simulink library "speedgoatlib_evse"  (R2024b)
settings: Solver=VariableStepAuto  StartTime=0.0  StopTime=10.0  RelTol=1e-3
undefined symbols (not defined in the file): sg_ev_charging_read_m, sg_ev_charging_write_m, sg_ev_isolation_read_m, sg_ev_parameter_read_m, sg_ev_parameter_write_m, sg_ev_precharge_read_m, sg_ev_precharge_write_m, sg_ev_status_m, sg_ev_stop_read_m, sg_ev_stop_write_m, sg_ev_welding_read_m, sg_ev_welding_write_m, sg_evse_charging_read_m, sg_evse_charging_write_m, sg_evse_isolation_read_m, sg_evse_isolation_write_m, sg_evse_parameter_read_m, sg_evse_parameter_write_m, sg_evse_precharge_read_m, sg_evse_precharge_write_m, sg_evse_status_m, sg_evse_stop_read_m, sg_evse_stop_write_m, sg_evse_welding_read_m, sg_evse_welding_write_m
libraries: speedgoatlib_mqtt x199, simulink x39, $bdroot x24
(part 1 of 8)
settings Model: Creator=timo.straessle  LastModifiedBy=speedgoat\jenkins
settings OptimizationCC: ReuseModelBlockBuffer=off
settings RTWCC: GPUComputeCapability=3.5
settings ConfigComp: CovBoundaryAbsTol=1.0e-5

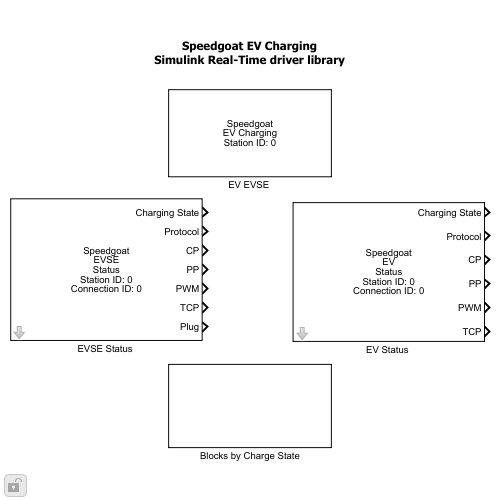
[thumbnail: Simulink's stored preview of the top-level diagram]
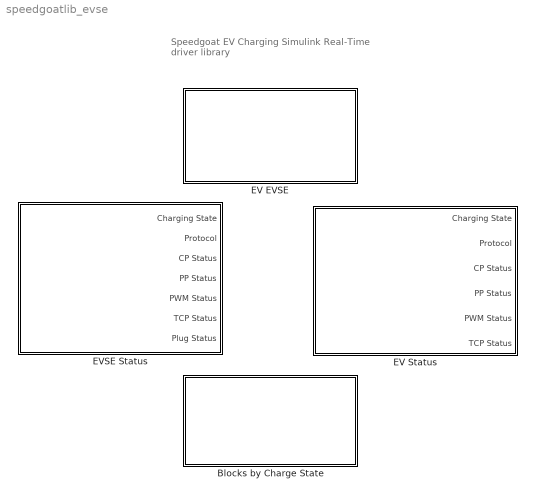
== system speedgoatlib_evse ==
  note: Speedgoat EV Charging
      | Simulink Real-Time driver library
  Blocks by Charge State : Subsystem
  "EV EVSE " : Subsystem  mask(EV_EVSE){}
      settings: OpenFcn=sg_evse.openFcnConfig;
      mask Help: eval('sg.utils.help.show(''io_main/refentry_ref_ev_evse'');')
      mask Display: disp('Speedgoat\nEV Charging\nStation ID: 0');
  "EV Status " : Subsystem  InitFcn=sg_ev_status_m.runInitFcn();  mask(status_EV){parClientId=0, parConnectionId=0, parSampleTime=-1}
      mask prompts: parClientId "Station ID"; parConnectionId "Connection ID"; parSampleTime "Sample Time"
      mask help: Speedgoat Driver Block<br>EV - Status<br><br>&copy; 2007 - 2026, Speedgoat GmbH, <a href="matlab: web('www.speedgoat.com','-browser');">www.speedgoat.com</a>
      mask init:
      | sg_ev_status_m.runMaskInit();
      mask Help: eval('sg.utils.help.show(''io_main/refentry_ref_ev_status'');')
      mask DialogControl Container6 Prompt: Main
      mask DialogControl Container3 Prompt: Connection Setup
      mask Display: disp('Speedgoat\nEV\nStatus\nStation ID: 0\nConnection ID: 0');port_label('output',1,'Charging State');port_label('output',2,'Protocol');port_label('output',3,'CP');port_label('output',4,'PP');port_label('output',5,'PWM');port_label('output',6,'TCP');
  "EVSE Status " : Subsystem  InitFcn=sg_evse_status_m.runInitFcn();  mask(status_EVSE){parClientId=0, parConnectionId=0, parSampleTime=-1}
      mask prompts: parClientId "Station ID"; parConnectionId "Connection ID"; parSampleTime "Sample Time"
      mask help: Speedgoat Driver Block<br>EVSE - Status<br><br>&copy; 2007 - 2026, Speedgoat GmbH, <a href="matlab: web('www.speedgoat.com','-browser');">www.speedgoat.com</a>
      mask init:
      | sg_evse_status_m.runMaskInit();
      mask Help: eval('sg.utils.help.show(''io_main/refentry_ref_evse_status'');')
      mask DialogControl Container6 Prompt: Main
      mask DialogControl Container3 Prompt: Connection Setup
      mask Display: disp('Speedgoat\nEVSE\nStatus\nStation ID: 0\nConnection ID: 0');port_label('output',1,'Charging State');port_label('output',2,'Protocol');port_label('output',3,'CP');port_label('output',4,'PP');port_label('output',5,'PWM');port_label('output',6,'TCP');port_label('output',7,'Plug');

== system speedgoatlib_evse/Blocks by Charge State ==
  note: EV
  note: EVSE
  "EV Charging Read " : Subsystem  InitFcn=sg_ev_charging_read_m.runInitFcn();  mask(charging_read_EV){parClientId=0, parConnectionId=0, parSampleTime=-1}
      mask prompts: parClientId "Station ID"; parConnectionId "Connection ID"; parSampleTime "Sample Time"
      mask help: Speedgoat Driver Block<br>EV - Charging<br><br>&copy; 2007 - 2026, Speedgoat GmbH, <a href="matlab: web('www.speedgoat.com','-browser');">www.speedgoat.com</a>
      mask init:
      | sg_ev_charging_read_m.runMaskInit();
      mask Help: eval('sg.utils.help.show(''io_main/refentry_ref_ev_charging_read'');')
      mask DialogControl Container6 Prompt: Main
      mask DialogControl Container3 Prompt: Connection Setup
      mask Display: disp('Speedgoat\nEV\nCharging\nRead\nStation ID: 0\nConnection ID: 0');port_label('output',1,'EVSE Present Voltage');port_label('output',2,'EVSE Present Current');port_label('output',3,'EVSE Current Limit Achieved');port_label('output',4,'EVSE Voltage Limit Achieved');port_label('output',5,'EVSE Power Limit Achieved');port_label('output',6,'EVSE Max Voltage Limit');port_label('output',7,'EVSE Max Current Limit');port_label('output',8,'EVSE Max Power Limit');
  "EV Charging Write " : Subsystem  InitFcn=sg_ev_charging_write_m.runInitFcn();  mask(charging_write_EV){parClientId=0, parConnectionId=0, parSampleTime=-1, parEnReadyToChargeState=on, parEnChargingProfileTupleId=on, parEnChargeReady=on, parEnErrorCode=on, parEnRessSoc=on, parEnTargetVoltage=on, parEnTargetCurrent=on, parEnBulkChargingComplete=on, parEnChargingComplete=on, parEnRemainingTimeToBulkSoc=on, parEnRemainingTimeToFullSoc=on}
      mask prompts: parClientId "Station ID"; parConnectionId "Connection ID"; parSampleTime "Sample Time"; parEnReadyToChargeState "Ready to Charge State"; parEnChargingProfileTupleId "Charging Profile Tuple ID"; parEnChargeReady "Charge Ready"; parEnErrorCode "Errorcode"; parEnRessSoc "RESS SOC"; parEnTargetVoltage "Target Voltage"; parEnTargetCurrent "Target Current"; parEnBulkChargingComplete "Bulk Charging Complete"; parEnChargingComplete "Charging Complete"; parEnRemainingTimeToBulkSoc "Remaining Time to Bulk SOC"; parEnRemainingTimeToFullSoc "Remaining Time to Full SOC"
      mask help: Speedgoat Driver Block<br>EV - Charging<br><br>&copy; 2007 - 2026, Speedgoat GmbH, <a href="matlab: web('www.speedgoat.com','-browser');">www.speedgoat.com</a>
      mask init:
      | sg_ev_charging_write_m.runMaskInit();
      mask Help: eval('sg.utils.help.show(''io_main/refentry_ref_ev_charging_write'');')
      mask DialogControl Container6 Prompt: Main
      mask DialogControl Container3 Prompt: Connection Setup
      mask DialogControl Container10 Prompt: Enable/Disable Signals
      mask Display: disp('Speedgoat\nEV\nCharging\nWrite\nStation ID: 0\nConnection ID: 0');port_label('input',1,'Ready to Charge State');port_label('input',2,'Charging Profile Tuple ID');port_label('input',3,'Charge Ready');port_label('input',4,'Errorcode');port_label('input',5,'RESS SOC');port_label('input',6,'Target Voltage');port_label('input',7,'Target Current');port_label('input',8,'Bulk Charging Complete');port_label('input',9,'Charging Complete');port_label('input',10,'Remaining Time to Bulk SOC');port_label('input',11,'Remaining Time to Full SOC');
  "EV Isolation Read " : Subsystem  InitFcn=sg_ev_isolation_read_m.runInitFcn();  mask(isolation_read_EV){parClientId=0, parConnectionId=0, parSampleTime=-1}
      mask prompts: parClientId "Station ID"; parConnectionId "Connection ID"; parSampleTime "Sample Time"
      mask help: Speedgoat Driver Block<br>EV - Isolation<br><br>&copy; 2007 - 2026, Speedgoat GmbH, <a href="matlab: web('www.speedgoat.com','-browser');">www.speedgoat.com</a>
      mask init:
      | sg_ev_isolation_read_m.runMaskInit();
      mask Help: eval('sg.utils.help.show(''io_main/refentry_ref_ev_isolation_read'');')
      mask DialogControl Container6 Prompt: Main
      mask DialogControl Container3 Prompt: Connection Setup
      mask Display: disp('Speedgoat\nEV\nIsolation\nRead\nStation ID: 0\nConnection ID: 0');port_label('output',1,'EVSE Processing');port_label('output',2,'EVSE Isolationstatus');port_label('output',3,'EVSE Statuscode');
  "EV Isolation Write " : Subsystem  InitFcn=sg_ev_precharge_write_m.runInitFcn();  mask(isolation_write_EV){parClientId=0, parConnectionId=0, parSampleTime=-1, parEnReady=on, parEnErrorCode=on, parEnRessSoc=on}
      mask prompts: parClientId "Station ID"; parConnectionId "Connection ID"; parSampleTime "Sample Time"; parEnReady "Ready"; parEnErrorCode "Errorcode"; parEnRessSoc "RESS SOC"
      mask help: Speedgoat Driver Block<br>EV - Isolation<br><br>&copy; 2007 - 2026, Speedgoat GmbH, <a href="matlab: web('www.speedgoat.com','-browser');">www.speedgoat.com</a>
      mask init:
      | sg_ev_isolation_write_m.runMaskInit();
      mask Help: eval('sg.utils.help.show(''io_main/refentry_ref_ev_isolation_write'');')
      mask DialogControl Container6 Prompt: Main
      mask DialogControl Container3 Prompt: Connection Setup
      mask DialogControl Container10 Prompt: Enable/Disable Signals
      mask Display: disp('Speedgoat\nEV\nIsolation\nWrite\nStation ID: 0\nConnection ID: 0');port_label('input',1,'Ready');port_label('input',2,'Errorcode');port_label('input',3,'RESS SOC');
  "EV Parameter Read " : Subsystem  InitFcn=sg_ev_parameter_read_m.runInitFcn();  mask(parameter_read_EV){parClientId=0, parConnectionId=0, parSampleTime=-1}
      mask prompts: parClientId "Station ID"; parConnectionId "Connection ID"; parSampleTime "Sample Time"
      mask help: Speedgoat Driver Block<br>EV - Parameter Discovery<br><br>&copy; 2007 - 2026, Speedgoat GmbH, <a href="matlab: web('www.speedgoat.com','-browser');">www.speedgoat.com</a>
      mask init:
      | sg_ev_parameter_read_m.runMaskInit();
      mask Help: eval('sg.utils.help.show(''io_main/refentry_ref_ev_parameter_read'');')
      mask DialogControl Container6 Prompt: Main
      mask DialogControl Container3 Prompt: Connection Setup
      mask Display: disp('Speedgoat\nEV\nParameter Discovery\nRead\nStation ID: 0\nConnection ID: 0');port_label('output',1,'SA-Schedule: ID');port_label('output',2,'SA-Schedule: Start');port_label('output',3,'SA-Schedule: Duration');port_label('output',4,'SA-Schedule: PMax');port_label('output',5,'EVSE Max Voltage Limit');port_label('output',6,'EVSE Max Current Limit');port_label('output',7,'EVSE Max Power Limit');port_label('output',8,'EVSE Min Current Limit');port_label('output',9,'EVSE Min Voltage Limit');port_label('output',10,'EVSE Current Regulation Tolerance');port_label('output',11,'EVSE Peak Current Ripple');port_label('output',12,'EVSE Energy to be Delivered');port_label('output',13,'EVSE Notification Max Delay');port_label('output',14,'EVSE Notification');port_label('output',15,'EVSE Isolationstatus');port_label('output',16,'EVSE Statuscode');
  "EV Parameter Write " : Subsystem  InitFcn=sg_ev_parameter_write_m.runInitFcn();  mask(parameter_write_EV){parClientId=0, parConnectionId=0, parSampleTime=-1, parEnRequestedEnergyType=on, parEnDepartureTime=on, parEnMaxVoltageLimit=on, parEnMaxCurrentLimit=on, parEnMinCurrentLimit=on, parEnMaxPowerLimit=on, parEnReady=on, parEnErrorcode=on, parEnRessSoc=on, parEnEnergyCapacity=on, parEnEnergyRequest=on, parEnFullSoc=on, parEnBulkSoc=on}
      mask prompts: parClientId "Station ID"; parConnectionId "Connection ID"; parSampleTime "Sample Time"; parEnRequestedEnergyType "Requested Energy Type"; parEnDepartureTime "Departure Time"; parEnMaxVoltageLimit "Max Voltage Limit"; parEnMaxCurrentLimit "Max Current Limit"; parEnMinCurrentLimit "Min Current Limit"; parEnMaxPowerLimit "Max Power Limit"; parEnReady "Ready"; parEnErrorcode "Errorcode"; parEnRessSoc "RESS SOC"; parEnEnergyCapacity "Energy Capacity"; parEnEnergyRequest "Energy Request"; parEnFullSoc "Full SOC"; parEnBulkSoc "Bulk SOC"
      mask help: Speedgoat Driver Block<br>EV - Parameter Discovery<br><br>&copy; 2007 - 2026, Speedgoat GmbH, <a href="matlab: web('www.speedgoat.com','-browser');">www.speedgoat.com</a>
      mask init:
      | sg_ev_parameter_write_m.runMaskInit();
      mask Help: eval('sg.utils.help.show(''io_main/refentry_ref_ev_parameter_write'');')
      mask DialogControl Container6 Prompt: Main
      mask DialogControl Container3 Prompt: Connection Setup
      mask DialogControl Container10 Prompt: Enable/Disable Signals
      mask DialogControl Control2 Prompt: Uncheck unused signals to disable them and avoid sending out zeroes.
      mask Display: disp('Speedgoat\nEV\nParameter Discovery\nWrite\nStation ID: 0\nConnection ID: 0');port_label('input',1,'Requested Energy Type');port_label('input',2,'Departure Time');port_label('input',3,'Max Voltage Limit');port_label('input',4,'Max Current Limit');port_label('input',5,'Min Current Limit');port_label('input',6,'Max Power Limit');port_label('input',7,'Ready');port_label('input',8,'Errorcode');port_label('input',9,'RESS SOC');port_label('input',10,'Energy Capacity');port_label('input',11,'Energy Request');port_label('input',12,'Full SOC');port_label('input',13,'Bulk SOC');
  "EV Pre-Charge Read " : Subsystem  InitFcn=sg_ev_precharge_read_m.runInitFcn();  mask(precharge_read_EV){parClientId=0, parConnectionId=0, parSampleTime=-1}
      mask prompts: parClientId "Station ID"; parConnectionId "Connection ID"; parSampleTime "Sample Time"
      mask help: Speedgoat Driver Block<br>EV - Pre-Charge<br><br>&copy; 2007 - 2026, Speedgoat GmbH, <a href="matlab: web('www.speedgoat.com','-browser');">www.speedgoat.com</a>
      mask init:
      | sg_ev_precharge_read_m.runMaskInit();
      mask Help: eval('sg.utils.help.show(''io_main/refentry_ref_ev_precharge_read'');')
      mask DialogControl Container6 Prompt: Main
      mask DialogControl Container3 Prompt: Connection Setup
      mask Display: disp('Speedgoat\nEV\nPre-Charge\nRead\nStation ID: 0\nConnection ID: 0');port_label('output',1,'EVSE Isolationstatus');port_label('output',2,'EVSE Statuscode');port_label('output',3,'EVSE Present Voltage');
  "EV Pre-Charge Write " : Subsystem  InitFcn=sg_ev_precharge_write_m.runInitFcn();  mask(precharge_write_EV){parClientId=0, parConnectionId=0, parSampleTime=-1, parEnReady=on, parEnErrorCode=on, parEnRessSoc=on, parEnTargetVoltage=on, parEnTargetCurrent=on}
      mask prompts: parClientId "Station ID"; parConnectionId "Connection ID"; parSampleTime "Sample Time"; parEnReady "Ready"; parEnErrorCode "Errorcode"; parEnRessSoc "RESS SOC"; parEnTargetVoltage "Target Voltage"; parEnTargetCurrent "Target Current"
      mask help: Speedgoat Driver Block<br>EV - Pre-Charge<br><br>&copy; 2007 - 2026, Speedgoat GmbH, <a href="matlab: web('www.speedgoat.com','-browser');">www.speedgoat.com</a>
      mask init:
      | sg_ev_precharge_write_m.runMaskInit();
      mask Help: eval('sg.utils.help.show(''io_main/refentry_ref_ev_precharge_write'');')
      mask DialogControl Container6 Prompt: Main
      mask DialogControl Container3 Prompt: Connection Setup
      mask DialogControl Container10 Prompt: Enable/Disable Signals
      mask Display: disp('Speedgoat\nEV\nPre-Charge\nWrite\nStation ID: 0\nConnection ID: 0');port_label('input',1,'Ready');port_label('input',2,'Errorcode');port_label('input',3,'RESS SOC');port_label('input',4,'Target Voltage');port_label('input',5,'Target Current');
  "EV Setup " : Subsystem  mask(setup_EV){parClientId=0, parConnectionId=0, parClientIdentifier='speedgoat', parIpAddrStr='192.168.10.7', parSampleTime=-1, parTcpPort=1883, parRemoteIpAddrStr='192.168.10.9', parDepartureTime=3600*4, parMaxVoltageLimit=480, parMaxCurrentLimit=100, parMinCurrentLimit=5, parMaxPowerLimit=60000, parRessSoc=30, parEnergyCapacity=80000, parEnergyRequest=30000, parFullSoc=100, parBulkSoc=80}
      mask prompts: parClientId "Station ID"; parConnectionId "Connection ID"; parClientIdentifier "Client Identifier"; parIpAddrStr "Local IP Address"; parSampleTime "Sample Time"; parTcpPort "Remote TCP Port"; parRemoteIpAddrStr "Remote IP Address"; parDepartureTime "Departure Time [s]"; parMaxVoltageLimit "Max. Voltage Limit [V]"; parMaxCurrentLimit "Max. Current Limit [A]"; parMinCurrentLimit "Min. Current Limit [A]"; parMaxPowerLimit "Max. Power Limit [W]"; parRessSoc "RESS SOC"; parEnergyCapacity "Energy Capacity [Wh]"; parEnergyRequest "Energy Request [Wh]"; parFullSoc "Full SOC"; parBulkSoc "Bulk SOC"
      mask Help: eval('sg.utils.help.show(''io_main/refentry_ref_ev_setup'');')
      mask TypeOptions parDepartureTime: departureTime/Value
      mask TypeOptions parMaxVoltageLimit: maxVoltageLimit/Value
      mask TypeOptions parMaxCurrentLimit: maxCurrentLimit/Value
      mask TypeOptions parMinCurrentLimit: minCurrentLimit/Value
      mask TypeOptions parMaxPowerLimit: maxPowerLimit/Value
      mask TypeOptions parRessSoc: ressSoc/Value
      mask TypeOptions parEnergyCapacity: energyCapacity/Value
      mask TypeOptions parEnergyRequest: energyRequest/Value
      mask TypeOptions parFullSoc: fullSoc/Value
      mask TypeOptions parBulkSoc: bulkSoc/Value
      mask DialogControl Container6 Prompt: Main
      mask DialogControl Container3 Prompt: Connection Setup
      mask DialogControl Container8 Prompt: EV Board Setup
      mask DialogControl Container10 Prompt: Vehicle Configuration Parameters
      mask Display: disp('Speedgoat\nEV Setup\n');
  "EV Stop Read " : Subsystem  InitFcn=sg_ev_stop_read_m.runInitFcn();  mask(stop_read_EV){parClientId=0, parConnectionId=0, parSampleTime=-1}
      mask prompts: parClientId "Station ID"; parConnectionId "Connection ID"; parSampleTime "Sample Time"
      mask help: Speedgoat Driver Block<br>EV - Stop<br><br>&copy; 2007 - 2026, Speedgoat GmbH, <a href="matlab: web('www.speedgoat.com','-browser');">www.speedgoat.com</a>
      mask init:
      | sg_ev_stop_read_m.runMaskInit();
      mask Help: eval('sg.utils.help.show(''io_main/refentry_ref_ev_stop_read'');')
      mask DialogControl Container6 Prompt: Main
      mask DialogControl Container3 Prompt: Connection Setup
      mask Display: disp('Speedgoat\nEV\nStop\nRead\nStation ID: 0\nConnection ID: 0');port_label('output',1,'EVSE Stop Progress');port_label('output',2,'EVSE Processing');
  "EV Stop Write " : Subsystem  InitFcn=sg_ev_stop_write_m.runInitFcn();  mask(stop_write_EV){parClientId=0, parConnectionId=0, parSampleTime=-1, parEnStopProgress=on}
      mask prompts: parClientId "Station ID"; parConnectionId "Connection ID"; parSampleTime "Sample Time"; parEnStopProgress "Stop Progress"
      mask help: Speedgoat Driver Block<br>EV - Stop<br><br>&copy; 2007 - 2026, Speedgoat GmbH, <a href="matlab: web('www.speedgoat.com','-browser');">www.speedgoat.com</a>
      mask init:
      | sg_ev_stop_write_m.runMaskInit();
      mask Help: eval('sg.utils.help.show(''io_main/refentry_ref_ev_stop_write'');')
      mask DialogControl Container6 Prompt: Main
      mask DialogControl Container3 Prompt: Connection Setup
      mask DialogControl Container10 Prompt: Enable/Disable Signals
      mask Display: disp('Speedgoat\nEV\nStop\nWrite\nStation ID: 0\nConnection ID: 0');port_label('input',1,'Stop Progress');
  "EV Welding Read " : Subsystem  InitFcn=sg_ev_welding_read_m.runInitFcn();  mask(welding_read_EV){parClientId=0, parConnectionId=0, parSampleTime=-1}
      mask prompts: parClientId "Station ID"; parConnectionId "Connection ID"; parSampleTime "Sample Time"
      mask help: Speedgoat Driver Block<br>EV - Welding<br><br>&copy; 2007 - 2026, Speedgoat GmbH, <a href="matlab: web('www.speedgoat.com','-browser');">www.speedgoat.com</a>
      mask init:
      | sg_ev_welding_read_m.runMaskInit();
      mask Help: eval('sg.utils.help.show(''io_main/refentry_ref_ev_welding_read'');')
      mask DialogControl Container6 Prompt: Main
      mask DialogControl Container3 Prompt: Connection Setup
      mask Display: disp('Speedgoat\nEV\nWelding\nRead\nStation ID: 0\nConnection ID: 0');port_label('output',1,'EVSE Notification');port_label('output',2,'EVSE Isolationstatus');port_label('output',3,'EVSE Statuscode');port_label('output',4,'EVSE Present Voltage');
  "EV Welding Write " : Subsystem  InitFcn=sg_ev_welding_write_m.runInitFcn();  mask(welding_write_EV){parClientId=0, parConnectionId=0, parSampleTime=-1, parEnReady=on, parEnErrorCode=on, parEnRessSoc=on}
      mask prompts: parClientId "Station ID"; parConnectionId "Connection ID"; parSampleTime "Sample Time"; parEnReady "Ready"; parEnErrorCode "Errorcode"; parEnRessSoc "RESS SOC"
      mask help: Speedgoat Driver Block<br>EV - Welding<br><br>&copy; 2007 - 2026, Speedgoat GmbH, <a href="matlab: web('www.speedgoat.com','-browser');">www.speedgoat.com</a>
      mask init:
      | sg_ev_welding_write_m.runMaskInit();
      mask Help: eval('sg.utils.help.show(''io_main/refentry_ref_ev_welding_write'');')
      mask DialogControl Container6 Prompt: Main
      mask DialogControl Container3 Prompt: Connection Setup
      mask DialogControl Container10 Prompt: Enable/Disable Signals
      mask Display: disp('Speedgoat\nEV\nWelding\nWrite\nStation ID: 0\nConnection ID: 0');port_label('input',1,'Ready');port_label('input',2,'Errorcode');port_label('input',3,'RESS SOC');
  "EVSE Charging Read " : Subsystem  InitFcn=sg_evse_charging_read_m.runInitFcn();  mask(charging_read_EVSE){parClientId=0, parConnectionId=0, parSampleTime=-1}
      mask prompts: parClientId "Station ID"; parConnectionId "Connection ID"; parSampleTime "Sample Time"
      mask help: Speedgoat Driver Block<br>EVSE - Charging<br><br>&copy; 2007 - 2026, Speedgoat GmbH, <a href="matlab: web('www.speedgoat.com','-browser');">www.speedgoat.com</a>
      mask init:
      | sg_evse_charging_read_m.runMaskInit();
      mask Help: eval('sg.utils.help.show(''io_main/refentry_ref_evse_charging_read'');')
      mask DialogControl Container6 Prompt: Main
      mask DialogControl Container3 Prompt: Connection Setup
      mask Display: disp('Speedgoat\nEVSE\nCharging\nRead\nStation ID: 0\nConnection ID: 0');port_label('output',1,'EV Ready');port_label('output',2,'EV Errorcode');port_label('output',3,'EV RESS SOC');port_label('output',4,'EV Target Voltage');port_label('output',5,'EV Target Current');port_label('output',6,'EV Max Voltage Limit');port_label('output',7,'EV Max Current Limit');port_label('output',8,'EV Max Power Limit');port_label('output',9,'EV Bulk Charging Complete');port_label('output',10,'EV Charging Complete');port_label('output',11,'EV Time to Bulk SOC');port_label('output',12,'EV Time to Full SOC');
  "EVSE Charging Write " : Subsystem  InitFcn=sg_evse_charging_write_m.runInitFcn();  mask(charging_write_EVSE){parClientId=0, parConnectionId=0, parSampleTime=-1, parEnNotification=on, parEnIsolationStatus=on, parEnStatusCode=on, parEnPresentVoltage=on, parEnPresentCurrent=on, parEnCurrentLimitAchieved=on, parEnVoltageLimitAchieved=on, parEnPowerLimitAchieved=on, parEnMaxVoltageLimit=on, parEnMaxCurrentLimit=on, parEnMaxPowerLimit=on}
      mask prompts: parClientId "Station ID"; parConnectionId "Connection ID"; parSampleTime "Sample Time"; parEnNotification "Notification"; parEnIsolationStatus "Isolationstatus"; parEnStatusCode "Statuscode"; parEnPresentVoltage "Present Voltage"; parEnPresentCurrent "Present Current"; parEnCurrentLimitAchieved "Current Limit Achieved"; parEnVoltageLimitAchieved "Voltage Limit Achieved"; parEnPowerLimitAchieved "Power Limit Achieved"; parEnMaxVoltageLimit "Max Voltage Limit"; parEnMaxCurrentLimit "Max Current Limit"; parEnMaxPowerLimit "Max Power Limit"
      mask help: Speedgoat Driver Block<br>EVSE - Charging<br><br>&copy; 2007 - 2026, Speedgoat GmbH, <a href="matlab: web('www.speedgoat.com','-browser');">www.speedgoat.com</a>
      mask init:
      | sg_evse_charging_write_m.runMaskInit();
      mask Help: eval('sg.utils.help.show(''io_main/refentry_ref_evse_charging_write'');')
      mask DialogControl Container6 Prompt: Main
      mask DialogControl Container3 Prompt: Connection Setup
      mask DialogControl Container10 Prompt: Enable/Disable Signals
      mask Display: disp('Speedgoat\nEVSE\nCharging\nWrite\nStation ID: 0\nConnection ID: 0');port_label('input',1,'Notification');port_label('input',2,'Isolationstatus');port_label('input',3,'Statuscode');port_label('input',4,'Present Voltage');port_label('input',5,'Present Current');port_label('input',6,'Current Limit Achieved');port_label('input',7,'Voltage Limit Achieved');port_label('input',8,'Power Limit Achieved');port_label('input',9,'Max Voltage Limit');port_label('input',10,'Max Current Limit');port_label('input',11,'Max Power Limit');
  "EVSE Isolation Read " : Subsystem  InitFcn=sg_evse_isolation_read_m.runInitFcn();  mask(isolation_read_EVSE){parClientId=0, parConnectionId=0, parSampleTime=-1}
      mask prompts: parClientId "Station ID"; parConnectionId "Connection ID"; parSampleTime "Sample Time"
      mask help: Speedgoat Driver Block<br>EVSE - Isolation<br><br>&copy; 2007 - 2026, Speedgoat GmbH, <a href="matlab: web('www.speedgoat.com','-browser');">www.speedgoat.com</a>
      mask init:
      | sg_evse_isolation_read_m.runMaskInit();
      mask Help: eval('sg.utils.help.show(''io_main/refentry_ref_evse_isolation_read'');')
      mask DialogControl Container6 Prompt: Main
      mask DialogControl Container3 Prompt: Connection Setup
      mask Display: disp('Speedgoat\nEVSE\nIsolation\nRead\nStation ID: 0\nConnection ID: 0');port_label('output',1,'EV Ready');port_label('output',2,'EV Errorcode');port_label('output',3,'EV RESS SOC');
  "EVSE Isolation Write " : Subsystem  InitFcn=sg_evse_isolation_write_m.runInitFcn();  mask(isolation_write_EVSE){parClientId=0, parConnectionId=0, parSampleTime=-1, parEnEvseProcessing=on, parEnIsolationStatus=on, parEnStatusCode=on}
      mask prompts: parClientId "Station ID"; parConnectionId "Connection ID"; parSampleTime "Sample Time"; parEnEvseProcessing "EVSE Processing"; parEnIsolationStatus "Isolationstatus"; parEnStatusCode "Statuscode"
      mask help: Speedgoat Driver Block<br>EVSE - Isolation<br><br>&copy; 2007 - 2026, Speedgoat GmbH, <a href="matlab: web('www.speedgoat.com','-browser');">www.speedgoat.com</a>
      mask init:
      | sg_evse_isolation_write_m.runMaskInit();
      mask Help: eval('sg.utils.help.show(''io_main/refentry_ref_evse_isolation_write'');')
      mask DialogControl Container6 Prompt: Main
      mask DialogControl Container3 Prompt: Connection Setup
      mask DialogControl Container10 Prompt: Enable/Disable Signals
      mask Display: disp('Speedgoat\nEVSE\nIsolation\nWrite\nStation ID: 0\nConnection ID: 0');port_label('input',1,'EVSE Processing');port_label('input',2,'Isolationstatus');port_label('input',3,'Statuscode');
  "EVSE Parameter Read " : Subsystem  InitFcn=sg_evse_parameter_read_m.runInitFcn();  mask(parameter_read_EVSE){parClientId=0, parConnectionId=0, parSampleTime=-1}
      mask prompts: parClientId "Station ID"; parConnectionId "Connection ID"; parSampleTime "Sample Time"
      mask help: Speedgoat Driver Block<br>EVSE - Parameter Discovery<br><br>&copy; 2007 - 2026, Speedgoat GmbH, <a href="matlab: web('www.speedgoat.com','-browser');">www.speedgoat.com</a>
      mask init:
      | sg_evse_parameter_read_m.runMaskInit();
      mask Help: eval('sg.utils.help.show(''io_main/refentry_ref_evse_parameter_read'');')
      mask DialogControl Container6 Prompt: Main
      mask DialogControl Container3 Prompt: Connection Setup
      mask Display: disp('Speedgoat\nEVSE\nParameter Discovery\nRead\nStation ID: 0\nConnection ID: 0');port_label('output',1,'EV Requested Energy Type');port_label('output',2,'EV Departure Time');port_label('output',3,'EV Max Voltage Limit');port_label('output',4,'EV Max Current Limit');port_label('output',5,'EV Min Current Limit');port_label('output',6,'EV Max Power Limit');port_label('output',7,'EV Ready');port_label('output',8,'EV Errorcode');port_label('output',9,'EV RESS SOC');port_label('output',10,'EV Energy Capacity');port_label('output',11,'EV Energy Request');port_label('output',12,'EV Full SOC');port_label('output',13,'EV Bulk SOC');
  "EVSE Parameter Write " : Subsystem  InitFcn=sg_evse_parameter_write_m.runInitFcn();  mask(parameter_write_EVSE){parClientId=0, parConnectionId=0, parSampleTime=-1, parEnEvseProcessing=on, parEnSaScheduleList=on, parEnMaxVoltageLimit=on, parEnMaxCurrentLimit=on, parEnMaxPowerLimit=on, parEnMinVoltageLimit=on, parEnMinCurrentLimit=on, parEnCurrRegTol=on, parEnPeakCurrentRipple=on, parEnEnergyToBeDelivered=on, parEnNotificationMaxDelay=on, parEnNotification=on, parEnIsolationStatus=on, parEnStatusCode=on}
      mask prompts: parClientId "Station ID"; parConnectionId "Connection ID"; parSampleTime "Sample Time"; parEnEvseProcessing "EVSE Processing"; parEnSaScheduleList "SA-Schedule List"; parEnMaxVoltageLimit "Max Voltage Limit"; parEnMaxCurrentLimit "Max Current Limit"; parEnMaxPowerLimit "Max Power Limit"; parEnMinVoltageLimit "Min Voltage Limit"; parEnMinCurrentLimit "Min Current Limit"; parEnCurrRegTol "Current Regulation Tolerance"; parEnPeakCurrentRipple "Peak Current Ripple"; parEnEnergyToBeDelivered "Energy To Be Delivered"; parEnNotificationMaxDelay "Notification Max Delay"; parEnNotification "Notification"; parEnIsolationStatus "Isolationstatus"; parEnStatusCode "Statuscode"
      mask help: Speedgoat Driver Block<br>EVSE - Parameter Discovery<br><br>&copy; 2007 - 2026, Speedgoat GmbH, <a href="matlab: web('www.speedgoat.com','-browser');">www.speedgoat.com</a>
      mask init:
      | sg_evse_parameter_write_m.runMaskInit();
      mask Help: eval('sg.utils.help.show(''io_main/refentry_ref_evse_parameter_write'');')
      mask DialogControl Container6 Prompt: Main
      mask DialogControl Container3 Prompt: Connection Setup
      mask DialogControl Container10 Prompt: Enable/Disable Signals
      mask DialogControl Control2 Prompt: Uncheck unused signals to disable them and avoid sending out zeroes.
      mask Display: disp('Speedgoat\nEVSE\nParameter Discovery\nWrite\nStation ID: 0\nConnection ID: 0');port_label('input',1,'EVSE Processing');port_label('input',2,'SA-Schedule: ID');port_label('input',3,'SA-Schedule: Start');port_label('input',4,'SA-Schedule: Duration');port_label('input',5,'SA-Schedule: PMax');port_label('input',6,'Max Voltage Limit');port_label('input',7,'Max Current Limit');port_label('input',8,'Max Power Limit');port_label('input',9,'Min Voltage Limit');port_label('input',10,'Min Current Limit');port_label('input',11,'Current Regulation Tolerance');port_label('input',12,'Peak Current Ripple');port_label('input',13,'Energy to be Delivered');port_label('input',14,'Notification Max Delay');port_label('input',15,'Notification');port_label('input',16,'Isolationstatus');port_label('input',17,'Statuscode');
  "EVSE Pre-Charge Read " : Subsystem  InitFcn=sg_evse_precharge_read_m.runInitFcn();  mask(precharge_read_EVSE){parClientId=0, parConnectionId=0, parSampleTime=-1}
      mask prompts: parClientId "Station ID"; parConnectionId "Connection ID"; parSampleTime "Sample Time"
      mask help: Speedgoat Driver Block<br>EVSE - Pre-Charge<br><br>&copy; 2007 - 2026, Speedgoat GmbH, <a href="matlab: web('www.speedgoat.com','-browser');">www.speedgoat.com</a>
      mask init:
      | sg_evse_precharge_read_m.runMaskInit();
      mask Help: eval('sg.utils.help.show(''io_main/refentry_ref_evse_precharge_read'');')
      mask DialogControl Container6 Prompt: Main
      mask DialogControl Container3 Prompt: Connection Setup
      mask Display: disp('Speedgoat\nEVSE\nPre-Charge\nRead\nStation ID: 0\nConnection ID: 0');port_label('output',1,'EV Ready');port_label('output',2,'EV Errorcode');port_label('output',3,'EV RESS SOC');port_label('output',4,'EV Target Voltage');port_label('output',5,'EV Target Current');
  "EVSE Pre-Charge Write " : Subsystem  InitFcn=sg_evse_precharge_write_m.runInitFcn();  mask(precharge_write_EVSE){parClientId=0, parConnectionId=0, parSampleTime=-1, parEnIsolationStatus=on, parEnStatusCode=on, parEnPresentVoltage=on}
      mask prompts: parClientId "Station ID"; parConnectionId "Connection ID"; parSampleTime "Sample Time"; parEnIsolationStatus "Isolationstatus"; parEnStatusCode "Statuscode"; parEnPresentVoltage "Present Voltage"
      mask help: Speedgoat Driver Block<br>EVSE - Pre-Charge<br><br>&copy; 2007 - 2026, Speedgoat GmbH, <a href="matlab: web('www.speedgoat.com','-browser');">www.speedgoat.com</a>
      mask init:
      | sg_evse_precharge_write_m.runMaskInit();
      mask Help: eval('sg.utils.help.show(''io_main/refentry_ref_evse_precharge_write'');')
      mask DialogControl Container6 Prompt: Main
      mask DialogControl Container3 Prompt: Connection Setup
      mask DialogControl Container10 Prompt: Enable/Disable Signals
      mask Display: disp('Speedgoat\nEVSE\nPre-Charge\nWrite\nStation ID: 0\nConnection ID: 0');port_label('input',1,'Isolationstatus');port_label('input',2,'Statuscode');port_label('input',3,'Present Voltage');
  "EVSE Setup " : Subsystem  mask(setup_EVSE){parClientId=0, parConnectionId=0, parClientIdentifier='speedgoat', parIpAddrStr='192.168.10.7', parSampleTime=-1, parTcpPort=1883, parRemoteIpAddrStr='192.168.10.8', parMaxVoltageLimit=480, parMaxCurrentLimit=100, parMinCurrentLimit=5, parMaxPowerLimit=60000, parMinVoltageLimit=12, parCurrRegTol=5, parPeakCurrentRipple=0}
      mask prompts: parClientId "Station ID"; parConnectionId "Connection ID"; parClientIdentifier "Client Identifier"; parIpAddrStr "Local IP Address"; parSampleTime "Sample Time"; parTcpPort "Remote TCP Port"; parRemoteIpAddrStr "Remote IP Address"; parMaxVoltageLimit "Max. Voltage Limit [V]"; parMaxCurrentLimit "Max. Current Limit [A]"; parMinCurrentLimit "Min. Current Limit [A]"; parMaxPowerLimit "Max. Power Limit [W]"; parMinVoltageLimit "Min. Voltage Limit [V]"; parCurrRegTol "Current Regulation Tolerance"; parPeakCurrentRipple "Peak Current Ripple"
      mask Help: eval('sg.utils.help.show(''io_main/refentry_ref_evse_setup'');')
      mask TypeOptions parMaxVoltageLimit: maxVoltageLimit/Value
      mask TypeOptions parMaxCurrentLimit: maxCurrentLimit/Value
      mask TypeOptions parMinCurrentLimit: minCurrentLimit/Value
      mask TypeOptions parMaxPowerLimit: maxPowerLimit/Value
      mask TypeOptions parMinVoltageLimit: minVoltageLimit/Value
      mask TypeOptions parCurrRegTol: currentRegulationTolerance/Value
      mask TypeOptions parPeakCurrentRipple: peakCurrentRipple/Value
      mask DialogControl Container6 Prompt: Main
      mask DialogControl Container3 Prompt: Connection Setup
      mask DialogControl Container8 Prompt: EVSE Board Setup
      mask DialogControl Container10 Prompt: Charging Configuration Parameters
      mask Display: disp('Speedgoat\nEVSE Setup\n');
  "EVSE Stop Read " : Subsystem  InitFcn=sg_evse_stop_read_m.runInitFcn();  mask(stop_read_EVSE){parClientId=0, parConnectionId=0, parSampleTime=-1}
      mask prompts: parClientId "Station ID"; parConnectionId "Connection ID"; parSampleTime "Sample Time"
      mask help: Speedgoat Driver Block<br>EVSE - Stop<br><br>&copy; 2007 - 2026, Speedgoat GmbH, <a href="matlab: web('www.speedgoat.com','-browser');">www.speedgoat.com</a>
      mask init:
      | sg_evse_stop_read_m.runMaskInit();
      mask Help: eval('sg.utils.help.show(''io_main/refentry_ref_evse_stop_read'');')
      mask DialogControl Container6 Prompt: Main
      mask DialogControl Container3 Prompt: Connection Setup
      mask Display: disp('Speedgoat\nEVSE\nStop\nRead\nStation ID: 0\nConnection ID: 0');port_label('output',1,'EV Stop Progress');
  "EVSE Stop Write " : Subsystem  InitFcn=sg_evse_stop_write_m.runInitFcn();  mask(stop_write_EVSE){parClientId=0, parConnectionId=0, parSampleTime=-1, parEnStopProgress=on, parEnEvseProcessing=on}
      mask prompts: parClientId "Station ID"; parConnectionId "Connection ID"; parSampleTime "Sample Time"; parEnStopProgress "Stop Progress"; parEnEvseProcessing "EVSE Processing"
      mask help: Speedgoat Driver Block<br>EVSE - Stop<br><br>&copy; 2007 - 2026, Speedgoat GmbH, <a href="matlab: web('www.speedgoat.com','-browser');">www.speedgoat.com</a>
      mask init:
      | sg_evse_stop_write_m.runMaskInit();
      mask Help: eval('sg.utils.help.show(''io_main/refentry_ref_evse_stop_write'');')
      mask DialogControl Container6 Prompt: Main
      mask DialogControl Container3 Prompt: Connection Setup
      mask DialogControl Container10 Prompt: Enable/Disable Signals
      mask Display: disp('Speedgoat\nEVSE\nStop\nWrite\nStation ID: 0\nConnection ID: 0');port_label('input',1,'Stop Progress');port_label('input',2,'EVSE Processing');
  "EVSE Welding Read " : Subsystem  InitFcn=sg_evse_welding_read_m.runInitFcn();  mask(welding_read_EVSE){parClientId=0, parConnectionId=0, parSampleTime=-1}
      mask prompts: parClientId "Station ID"; parConnectionId "Connection ID"; parSampleTime "Sample Time"
      mask help: Speedgoat Driver Block<br>EVSE - Welding<br><br>&copy; 2007 - 2026, Speedgoat GmbH, <a href="matlab: web('www.speedgoat.com','-browser');">www.speedgoat.com</a>
      mask init:
      | sg_evse_welding_read_m.runMaskInit();
      mask Help: eval('sg.utils.help.show(''io_main/refentry_ref_evse_welding_read'');')
      mask DialogControl Container6 Prompt: Main
      mask DialogControl Container3 Prompt: Connection Setup
      mask Display: disp('Speedgoat\nEVSE\nWelding\nRead\nStation ID: 0\nConnection ID: 0');port_label('output',1,'EV Ready');port_label('output',2,'EV Errorcode');port_label('output',3,'EV RESS SOC');
  "EVSE Welding Write " : Subsystem  InitFcn=sg_evse_welding_write_m.runInitFcn();  mask(welding_write_EVSE){parClientId=0, parConnectionId=0, parSampleTime=-1, parEnNotification=on, parEnIsolationStatus=on, parEnStatusCode=on, parEnPresentVoltage=on}
      mask prompts: parClientId "Station ID"; parConnectionId "Connection ID"; parSampleTime "Sample Time"; parEnNotification "Notification"; parEnIsolationStatus "Isolation Status"; parEnStatusCode "Statuscode"; parEnPresentVoltage "Present Voltage"
      mask help: Speedgoat Driver Block<br>EVSE - Welding<br><br>&copy; 2007 - 2026, Speedgoat GmbH, <a href="matlab: web('www.speedgoat.com','-browser');">www.speedgoat.com</a>
      mask init:
      | sg_evse_welding_write_m.runMaskInit();
      mask Help: eval('sg.utils.help.show(''io_main/refentry_ref_evse_welding_write'');')
      mask DialogControl Container6 Prompt: Main
      mask DialogControl Container3 Prompt: Connection Setup
      mask DialogControl Container10 Prompt: Enable/Disable Signals
      mask Display: disp('Speedgoat\nEVSE\nWelding\nWrite\nStation ID: 0\nConnection ID: 0');port_label('input',1,'Notification');port_label('input',2,'Isolationstatus');port_label('input',3,'Statuscode');port_label('input',4,'Present Voltage');

== system speedgoatlib_evse/EV EVSE  ==
  Subsystem : Subsystem

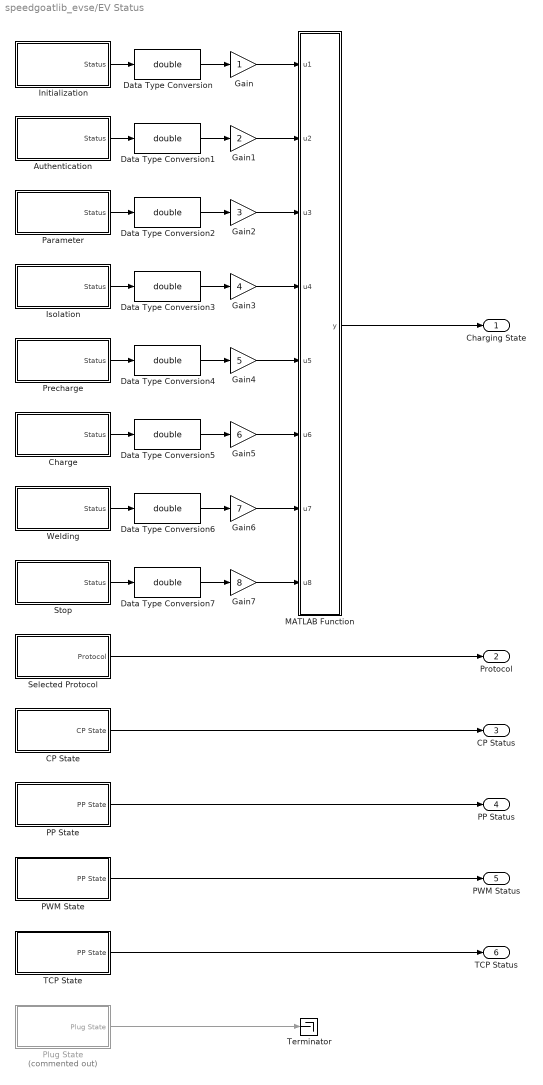
== system speedgoatlib_evse/EV Status  ==
  Authentication : Subsystem  VariantControl=Authentication State Status
  CP State : Subsystem  VariantControl=Stop State Status
  Charge : Subsystem  VariantControl=Charge State Status
  Data Type Conversion{,1..7} (8 alike) : DataTypeConversion  OutDataTypeStr=double  SaturateOnIntegerOverflow=off  RndMeth=Floor
  Gain : Gain
  Gain1 : Gain  Gain=2
  Gain2 : Gain  Gain=3
  Gain3 : Gain  Gain=4
  Gain4 : Gain  Gain=5
  Gain5 : Gain  Gain=6
  Gain6 : Gain  Gain=7
  Gain7 : Gain  Gain=8
  Initialization : Subsystem  VariantControl=Initialization State Status
  Isolation : Subsystem  VariantControl=Isolation State Status
  MATLAB Function : MATLAB Function  TreatAsAtomicUnit=on
  PP State : Subsystem  VariantControl=Stop State Status
  PWM State : Subsystem  VariantControl=Stop State Status
  Parameter : Subsystem  VariantControl=Parameter State Status
  Plug State : Subsystem  Commented=on  VariantControl=Stop State Status
  Precharge : Subsystem  VariantControl=Precharge State Status
  Selected Protocol : Subsystem  VariantControl=Stop State Status
  Stop : Subsystem  VariantControl=Stop State Status
  TCP State : Subsystem  VariantControl=Stop State Status
  Terminator : Terminator
  Welding : Subsystem  VariantControl=Welding State Status
  Charging State : Outport
  Protocol : Outport  Port=2
  CP Status : Outport  Port=3
  PP Status : Outport  Port=4
  PWM Status : Outport  Port=5
  TCP Status : Outport  Port=6
  wires:
  Data Type Conversion7/1 -> Gain7/1
  Data Type Conversion6/1 -> Gain6/1
  Data Type Conversion5/1 -> Gain5/1
  Data Type Conversion3/1 -> Gain3/1
  Data Type Conversion4/1 -> Gain4/1
  Data Type Conversion2/1 -> Gain2/1
  Data Type Conversion1/1 -> Gain1/1
  Data Type Conversion/1 -> Gain/1
  TCP State/1(PP State) -> TCP Status/1
  Plug State/1(Plug State) -> Terminator/1
  PWM State/1(PP State) -> PWM Status/1
  PP State/1(PP State) -> PP Status/1
  CP State/1(CP State) -> CP Status/1
  Selected Protocol/1(Protocol) -> Protocol/1
  Gain/1 -> MATLAB Function/1(u1)
  Gain1/1 -> MATLAB Function/2(u2)
  Gain2/1 -> MATLAB Function/3(u3)
  Gain3/1 -> MATLAB Function/4(u4)
  Gain4/1 -> MATLAB Function/5(u5)
  Gain5/1 -> MATLAB Function/6(u6)
  Gain6/1 -> MATLAB Function/7(u7)
  Gain7/1 -> MATLAB Function/8(u8)
  Precharge/1(Status) -> Data Type Conversion4/1
  Charge/1(Status) -> Data Type Conversion5/1
  Stop/1(Status) -> Data Type Conversion7/1
  Welding/1(Status) -> Data Type Conversion6/1
  Parameter/1(Status) -> Data Type Conversion2/1
  Isolation/1(Status) -> Data Type Conversion3/1
  Authentication/1(Status) -> Data Type Conversion1/1
  Initialization/1(Status) -> Data Type Conversion/1
  MATLAB Function/1(y) -> Charging State/1

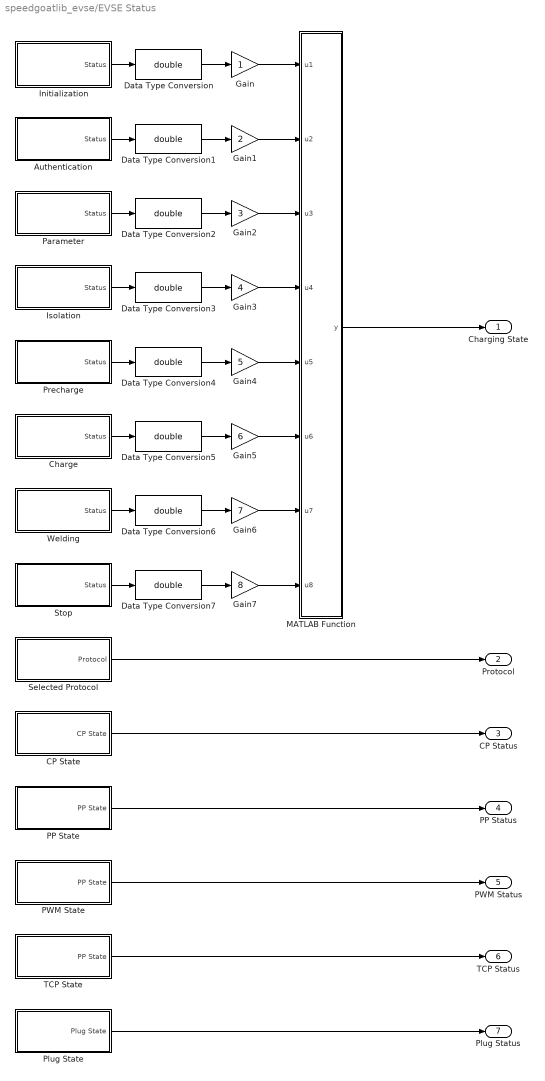
== system speedgoatlib_evse/EVSE Status  ==
  Authentication : Subsystem  VariantControl=Authentication State Status
  CP State : Subsystem  VariantControl=Stop State Status
  Charge : Subsystem  VariantControl=Charge State Status
  Data Type Conversion{,1..7} (8 alike) : DataTypeConversion  OutDataTypeStr=double  SaturateOnIntegerOverflow=off  RndMeth=Floor
  Gain : Gain
  Gain1 : Gain  Gain=2
  Gain2 : Gain  Gain=3
  Gain3 : Gain  Gain=4
  Gain4 : Gain  Gain=5
  Gain5 : Gain  Gain=6
  Gain6 : Gain  Gain=7
  Gain7 : Gain  Gain=8
  Initialization : Subsystem  VariantControl=Initialization State Status
  Isolation : Subsystem  VariantControl=Isolation State Status
  MATLAB Function : MATLAB Function  TreatAsAtomicUnit=on
  PP State : Subsystem  VariantControl=Stop State Status
  PWM State : Subsystem  VariantControl=Stop State Status
  Parameter : Subsystem  VariantControl=Parameter State Status
  Plug State : Subsystem  VariantControl=Stop State Status
  Precharge : Subsystem  VariantControl=Precharge State Status
  Selected Protocol : Subsystem  VariantControl=Stop State Status
  Stop : Subsystem  VariantControl=Stop State Status
  TCP State : Subsystem  VariantControl=Stop State Status
  Welding : Subsystem  VariantControl=Welding State Status
  Charging State : Outport
  Protocol : Outport  Port=2
  CP Status : Outport  Port=3
  PP Status : Outport  Port=4
  PWM Status : Outport  Port=5
  TCP Status : Outport  Port=6
  Plug Status : Outport  Port=7
  wires:
  MATLAB Function/1(y) -> Charging State/1
  Initialization/1(Status) -> Data Type Conversion/1
  Authentication/1(Status) -> Data Type Conversion1/1
  Isolation/1(Status) -> Data Type Conversion3/1
  Parameter/1(Status) -> Data Type Conversion2/1
  Welding/1(Status) -> Data Type Conversion6/1
  Stop/1(Status) -> Data Type Conversion7/1
  Charge/1(Status) -> Data Type Conversion5/1
  Precharge/1(Status) -> Data Type Conversion4/1
  Gain7/1 -> MATLAB Function/8(u8)
  Gain6/1 -> MATLAB Function/7(u7)
  Gain5/1 -> MATLAB Function/6(u6)
  Gain4/1 -> MATLAB Function/5(u5)
  Gain3/1 -> MATLAB Function/4(u4)
  Gain2/1 -> MATLAB Function/3(u3)
  Gain1/1 -> MATLAB Function/2(u2)
  Gain/1 -> MATLAB Function/1(u1)
  Selected Protocol/1(Protocol) -> Protocol/1
  CP State/1(CP State) -> CP Status/1
  PP State/1(PP State) -> PP Status/1
  PWM State/1(PP State) -> PWM Status/1
  Plug State/1(Plug State) -> Plug Status/1
  TCP State/1(PP State) -> TCP Status/1
  Data Type Conversion/1 -> Gain/1
  Data Type Conversion1/1 -> Gain1/1
  Data Type Conversion2/1 -> Gain2/1
  Data Type Conversion4/1 -> Gain4/1
  Data Type Conversion3/1 -> Gain3/1
  Data Type Conversion5/1 -> Gain5/1
  Data Type Conversion6/1 -> Gain6/1
  Data Type Conversion7/1 -> Gain7/1

== system speedgoatlib_evse/Blocks by Charge State/EV Charging Read  ==
  Charge Status Subscribe : speedgoatlib_mqtt/Client/MQTT Client Subscribe  ClientId=parClientId  ConnectionId=parConnectionId  Topic='port0/ci/charge/charge/status'  QoS=0 - at most once  InitValue=zeros(1,24,'uint8')  Extended=off  SampleTime=parSampleTime
      settings: SourceProductName=MQTT
  Compare To Constant : simulink/Logic and Bit Operations/Compare To Constant  relop===  const=1  OutDataTypeStr=boolean
  Enabled Subsystem : Subsystem  TreatAsAtomicUnit=on
  string compare logic1 : Subsystem
  evsePresentVoltage : Outport
  evsePresentCurrent : Outport  Port=2
  evseCurrentLimitAchieved : Outport  Port=3
  evseVoltageLimitAchieved : Outport  Port=4
  evsePowerLimitAchieved : Outport  Port=5
  evseMaxVoltageLimit : Outport  Port=6
  evseMaxCurrentLimit : Outport  Port=7
  evseMaxPowerLimit : Outport  Port=8
  wires:
  Charge Status Subscribe/1 -> string compare logic1/1(Input)
  string compare logic1/1(Out1) -> Compare To Constant/1
  Compare To Constant/1 -> Enabled Subsystem/Enable  "Charge State Reached"
  Enabled Subsystem/1(EVSE Present Voltage) -> evsePresentVoltage/1
  Enabled Subsystem/2(EVSE Present Current) -> evsePresentCurrent/1
  Enabled Subsystem/3(EVSE Current Limit Achieved) -> evseCurrentLimitAchieved/1
  Enabled Subsystem/4(EVSE Voltage Limit Achieved) -> evseVoltageLimitAchieved/1
  Enabled Subsystem/5(EVSE Power Limit Achieved) -> evsePowerLimitAchieved/1
  Enabled Subsystem/6(EVSE Max Voltage Limit) -> evseMaxVoltageLimit/1
  Enabled Subsystem/7(EVSE Max Current Limit) -> evseMaxCurrentLimit/1
  Enabled Subsystem/8(EVSE Max Power Limit) -> evseMaxPowerLimit/1

== system speedgoatlib_evse/Blocks by Charge State/EV Charging Write  ==
  readyToChargeState : Inport
  chargingProfileTupleId : Inport  Port=2
  chargeReady : Inport  Port=3
  errorCode : Inport  Port=4
  ressSoc : Inport  Port=5
  targetVoltage : Inport  Port=6
  targetCurrent : Inport  Port=7
  bulkChargingComplete : Inport  Port=8
  chargingComplete : Inport  Port=9
  remainingTimeToBulkSoc : Inport  Port=10
  remainingTimeToFullSoc : Inport  Port=11
  Charge Status Subscribe : speedgoatlib_mqtt/Client/MQTT Client Subscribe  ClientId=parClientId  ConnectionId=parConnectionId  Topic='port0/ci/charge/charge/status'  QoS=0 - at most once  InitValue=zeros(1,24,'uint8')  Extended=off  SampleTime=parSampleTime
      settings: SourceProductName=MQTT
  Compare To Constant : simulink/Logic and Bit Operations/Compare To Constant  relop===  const=1  OutDataTypeStr=boolean
  Compare To Constant1 : simulink/Logic and Bit Operations/Compare To Constant  relop===  const=1  OutDataTypeStr=boolean
  Compare To Constant2 : simulink/Logic and Bit Operations/Compare To Constant  relop===  const=1  OutDataTypeStr=boolean
  Enabled Subsystem : Subsystem  TreatAsAtomicUnit=on
  Enabled Subsystem1 : Subsystem  TreatAsAtomicUnit=on
  Isolation Status Subscribe : speedgoatlib_mqtt/Client/MQTT Client Subscribe  ClientId=parClientId  ConnectionId=parConnectionId  Topic='port0/ci/charge/isolation/status'  QoS=0 - at most once  InitValue=zeros(1,24,'uint8')  Extended=off  SampleTime=parSampleTime
      settings: SourceProductName=MQTT
  Logical Operator : Logic  Operator=OR  AllPortsSameDT=off  OutDataTypeStr=boolean
  OR : Logic  Operator=OR  Inputs=3  IconShape=distinctive  AllPortsSameDT=off  OutDataTypeStr=boolean
  Precharge Status Subscribe : speedgoatlib_mqtt/Client/MQTT Client Subscribe  ClientId=parClientId  ConnectionId=parConnectionId  Topic='port0/ci/charge/precharge/status'  QoS=0 - at most once  InitValue=zeros(1,24,'uint8')  Extended=off  SampleTime=parSampleTime
      settings: SourceProductName=MQTT
  string compare logic : Subsystem
  string compare logic1 : Subsystem
  string compare logic2 : Subsystem
  wires:
  remainingTimeToFullSoc/1 -> Enabled Subsystem/10(remainingtimetofullsoc)
  remainingTimeToBulkSoc/1 -> Enabled Subsystem/9(remainingtimetobulksoc)
  chargingComplete/1 -> Enabled Subsystem/8(chargingcomplete)
  bulkChargingComplete/1 -> Enabled Subsystem/7(bulkchargingcomplete)
  targetCurrent/1 -> Enabled Subsystem/6(targetcurrent)
  targetVoltage/1 -> Enabled Subsystem/5(targetvoltage)
  ressSoc/1 -> Enabled Subsystem/4(resssoc)
  chargeReady/1 -> Enabled Subsystem/2(chargeready)
  chargingProfileTupleId/1 -> Enabled Subsystem/1(chargingprofiletupleid)
  readyToChargeState/1 -> Enabled Subsystem1/1(readyToChargeState)
  OR/1 -> Enabled Subsystem1/Enable
  Compare To Constant1/1 -> Logical Operator/1, OR/2  "Precharge State Reached"
  Precharge Status Subscribe/1 -> string compare logic/1(Input)
  string compare logic/1(Out1) -> Compare To Constant1/1
  Compare To Constant/1 -> Logical Operator/2, OR/3  "Charge State Reached"
  string compare logic1/1(Out1) -> Compare To Constant/1
  Charge Status Subscribe/1 -> string compare logic1/1(Input)
  errorCode/1 -> Enabled Subsystem/3(errorcode)
  string compare logic2/1(Out1) -> Compare To Constant2/1
  Compare To Constant2/1 -> OR/1  "Isolation State Reached"
  Isolation Status Subscribe/1 -> string compare logic2/1(Input)
  Logical Operator/1 -> Enabled Subsystem/Enable

== system speedgoatlib_evse/Blocks by Charge State/EV Isolation Read  ==
  Compare To Constant : simulink/Logic and Bit Operations/Compare To Constant  relop===  const=1  OutDataTypeStr=boolean
  Enabled Subsystem : Subsystem  TreatAsAtomicUnit=on
  Isolation Status Subscribe : speedgoatlib_mqtt/Client/MQTT Client Subscribe  ClientId=parClientId  ConnectionId=parConnectionId  Topic='port0/ci/charge/isolation/status'  QoS=0 - at most once  InitValue=zeros(1,24,'uint8')  Extended=off  SampleTime=parSampleTime
      settings: SourceProductName=MQTT
  string compare logic1 : Subsystem
  evseProcessing : Outport
  evseIsolationstatus : Outport  Port=2
  evseStatuscode : Outport  Port=3
  wires:
  Isolation Status Subscribe/1 -> string compare logic1/1(Input)
  string compare logic1/1(Out1) -> Compare To Constant/1
  Compare To Constant/1 -> Enabled Subsystem/Enable  "Isolation State Reached"
  Enabled Subsystem/2(EVSE Isolationstatus) -> evseIsolationstatus/1
  Enabled Subsystem/3(EVSE Statuscode) -> evseStatuscode/1
  Enabled Subsystem/1(EVSE Processing) -> evseProcessing/1
